simulink model "CUSTOMPID"  (R2020b)
settings: Solver=FixedStepAuto  StartTime=0.0  StopTime=2  FixedStep=0.01  RelTol=1e-3
undefined symbols (not defined in the file): cont_tf5, DiscIntNeverNeededParam, sigbuilder_block, sysConverted, tf5
settings Model: DataTypeOverride=Off  FPTShortcutValueString='{{},{''BaselineRun'',1,1,1,''BaselineRun'','''',{},''M'','''',''''},{''BaselineRun_2'',1,1,1,''BaselineRun_2'','''',{},''M'','''',''''}}'  Creator=EMRE  LastModifiedBy=EMRE
settings SolverCC: AlgebraicLoopSolver=LineSearch
settings OptimizationCC: BlockReduction=off  ConditionallyExecuteInputs=off  DefaultParameterBehavior=Inlined
settings DebuggingCC: SignalRangeChecking=warning  AlgebraicLoopMsg=error  SingleTaskRateTransMsg=error
settings HardwareCC: ProdBitPerPointer=32  ProdBitPerSizeT=32  ProdBitPerPtrDiffT=32  ProdLargestAtomicFloat=None  ProdIntDivRoundTo=Undefined  ProdEndianess=Unspecified  ProdWordSize=32  ProdHWDeviceType=ASIC/FPGA->ASIC/FPGA  TargetBitPerPointer=64  TargetBitPerSizeT=64  TargetBitPerPtrDiffT=64  TargetLongLongMode=on  TargetIntDivRoundTo=Zero  TargetEndianess=LittleEndian  TargetWordSize=64  TargetHWDeviceType=Custom Processor->MATLAB Host Computer  ProdEqTarget=off

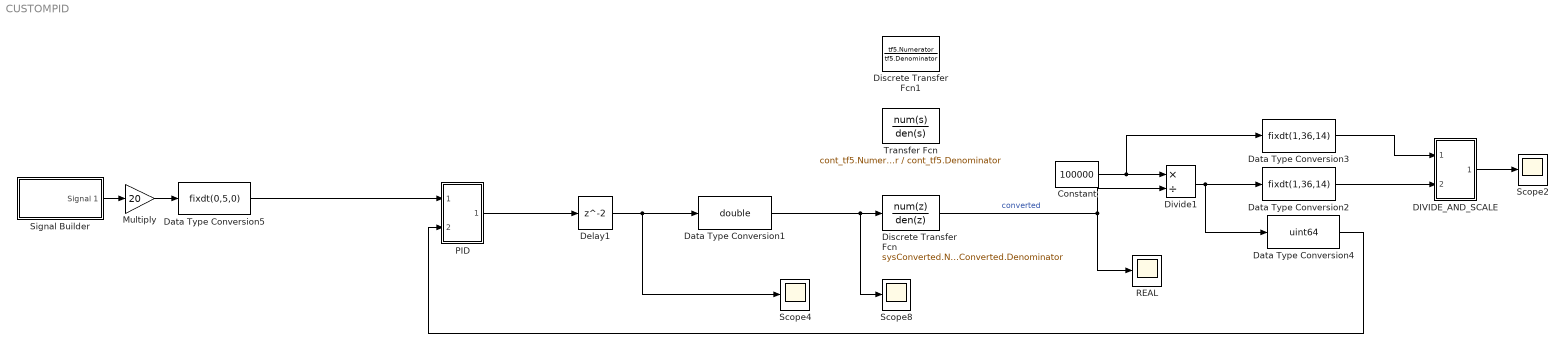
== system CUSTOMPID ==
  Constant : Constant  Value=100000
  DIVIDE_AND_SCALE : Subsystem
  Data Type Conversion1 : DataTypeConversion  OutDataTypeStr=double
  Data Type Conversion2 : DataTypeConversion  OutDataTypeStr=fixdt(1,36,14)
  Data Type Conversion3 : DataTypeConversion  OutDataTypeStr=fixdt(1,36,14)
  Data Type Conversion4 : DataTypeConversion  OutDataTypeStr=uint64  SaturateOnIntegerOverflow=on
  Data Type Conversion5 : DataTypeConversion  OutDataTypeStr=fixdt(0,5,0)
  Delay1 : Delay
  Discrete Transfer Fcn : DiscreteTransferFcn  Numerator=sysConverted.Numerator  Denominator=sysConverted.Denominator  InitialStates=1  SampleTime=0.01
  Discrete Transfer Fcn1 : DiscreteTransferFcn  Numerator=tf5.Numerator  Denominator=tf5.Denominator  SampleTime=1/100
  Divide1 : Product  Inputs=*/  RndMeth=Zero  SaturateOnIntegerOverflow=on
  Multiply : Gain  Gain=20
  PID : Subsystem
  REAL : Scope
  Scope2 : Scope
  Scope4 : Scope
  Scope8 : Scope
  Signal Builder : Subsystem  Tag=STV Subsys  LoadFcn=sigbuilder_block('load');  StartFcn=sigbuilder_block('start');  StopFcn=sigbuilder_block('stop');  ClipboardFcn=sigbuilder_block('clipboard');  mask(Sigbuilder block){tuvar=[0:10]}
      mask help: Simulink:masks:SigbuilderBlock_MD
      mask init:
      | if ~strcmp(get_param(bdroot(gcbh),'SimulationStatus'),'stopped') tuvar = sigbuilder_block('maskInit'); end
      settings: CopyFcn=sigbuilder_block('copy');  DeleteFcn=sigbuilder_block('delete');  ModelCloseFcn=sigbuilder_block('modelClose');  PreSaveFcn=sigbuilder_block('preSave');  PauseFcn=sigbuilder_block('pause');  ContinueFcn=sigbuilder_block('continue');  NameChangeFcn=sigbuilder_block('namechange');  OpenFcn=sigbuilder_block('open',[437.6 199.2 550.4 400 ]);  CloseFcn=sigbuilder_block('close');
      mask Display: plot(0, 0, 100, 100,[2, 2, 32, 32, 2], [68, 8, 8, 68, 68],[32, 2], [38, 38], [32, 19, 2],[53, 60, 44], [32, 17, 17, 2],[16, 16, 31, 31]);txt = getActiveGroup(gcbh);text(2, 100, txt,'verticalAlignment', 'top');
  Transfer Fcn : TransferFcn  Numerator=cont_tf5.Numerator  Denominator=cont_tf5.Denominator
  wires:
  Multiply/1 -> Data Type Conversion5/1
  Signal Builder/1(Signal 1) -> Multiply/1
  Discrete Transfer Fcn/1 -> REAL/1, Divide1/2  "converted"
  Data Type Conversion1/1 -> Discrete Transfer Fcn/1, Scope8/1
  Data Type Conversion2/1 -> DIVIDE_AND_SCALE/2(In2)
  Constant/1 -> Data Type Conversion3/1, Divide1/1
  DIVIDE_AND_SCALE/1(Out1) -> Scope2/1
  Data Type Conversion3/1 -> DIVIDE_AND_SCALE/1(In1)
  Divide1/1 -> Data Type Conversion4/1, Data Type Conversion2/1
  PID/1(Out1) -> Delay1/1
  Data Type Conversion5/1 -> PID/1(In1)
  Data Type Conversion4/1 -> PID/2(In2)
  Delay1/1 -> Data Type Conversion1/1, Scope4/1

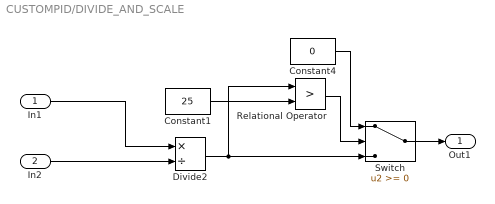
== system CUSTOMPID/DIVIDE_AND_SCALE ==
  In1 : Inport
  In2 : Inport  Port=2
  Constant1 : Constant  Value=25  OutDataTypeStr=fixdt(1,36,0)
  Constant4 : Constant  Value=0  OutDataTypeStr=fixdt(1,36,0)
  Divide2 : Product  Inputs=*/  OutMin=0  OutMax=25  OutDataTypeStr=fixdt(1,36,0)  RndMeth=Zero  SaturateOnIntegerOverflow=on
  Relational Operator : RelationalOperator  Operator=>  OutDataTypeStr=boolean  RndMeth=Simplest
  Switch : Switch  OutDataTypeStr=fixdt(1,36,0)
  Out1 : Outport
  wires:
  Switch/1 -> Out1/1
  Constant1/1 -> Relational Operator/2
  Constant4/1 -> Switch/1
  Relational Operator/1 -> Switch/2
  Divide2/1 -> Relational Operator/1, Switch/3
  In2/1 -> Divide2/2
  In1/1 -> Divide2/1

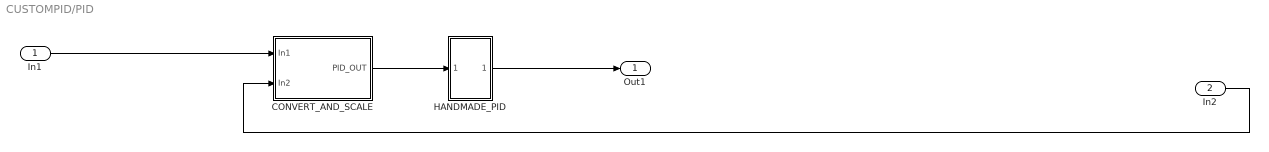
== system CUSTOMPID/PID ==
  In1 : Inport  SampleTime=1/100
  In2 : Inport  Port=2  SampleTime=1/100
  CONVERT_AND_SCALE : Subsystem
  HANDMADE_PID : Subsystem
  Out1 : Outport  SampleTime=1/100
  wires:
  CONVERT_AND_SCALE/1(PID_OUT) -> HANDMADE_PID/1(PID_OUT)
  HANDMADE_PID/1(Out1) -> Out1/1
  In1/1 -> CONVERT_AND_SCALE/1(In1)
  In2/1 -> CONVERT_AND_SCALE/2(In2)

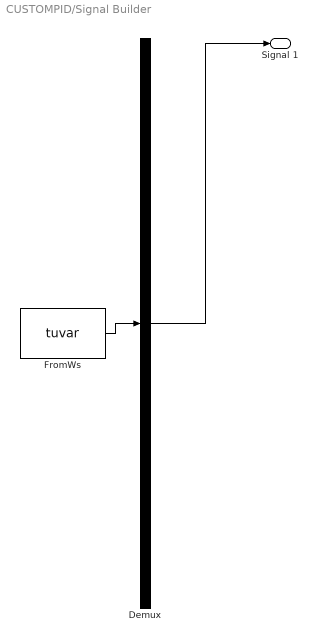
== system CUSTOMPID/Signal Builder ==
  Demux : Demux  Tag=STV Demux  Outputs=1
      settings: DisplayOption=none
  FromWs : FromWorkspace  Tag=STV FromWs  VariableName=tuvar
      SigBuilderData=|
      | common.afterFinalStr = 'Extrapolate'
      | common.sampleTime = 0
      | dataSet.timeRange = [0 2]
      | dataSet.name = 'Group 1'
      | sbobj.Groups.Name = 'Group 1'
      | sbobj.Groups.Signals.Name = 'Signal 1'
      | sbobj.Groups.Signals.XData = [0 0.2 0.5 0.7 0.7 1 1 1.1 1.1 1.3 1.3 1.4 1.4 1.5 1.5 1.7 1.7 2]
      | sbobj.Groups.Signals.YData = [1 1 1 1 0.2 0.195 0.99 0.99 0.2 0.2 0 0 0.4 0.4 0 0 1 1]
      | sbobj.Groups.TimeRange = [0 2]
  Signal 1 : Outport  Tag=STV Outport
  wires:
  Demux/1 -> Signal 1/1
  FromWs/1 -> Demux/1

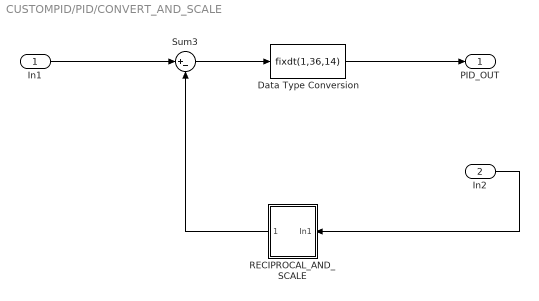
== system CUSTOMPID/PID/CONVERT_AND_SCALE ==
  In1 : Inport  SampleTime=1/100
  In2 : Inport  Port=2  SampleTime=1/100
  Data Type Conversion : DataTypeConversion  OutDataTypeStr=fixdt(1,36,14)
  RECIPROCAL_AND_SCALE : Subsystem
  Sum3 : Sum  Inputs=|+-
  PID_OUT : Outport  SampleTime=1/100
  wires:
  In1/1 -> Sum3/1
  RECIPROCAL_AND_SCALE/1(Out1) -> Sum3/2
  In2/1 -> RECIPROCAL_AND_SCALE/1(In1)
  Data Type Conversion/1 -> PID_OUT/1
  Sum3/1 -> Data Type Conversion/1

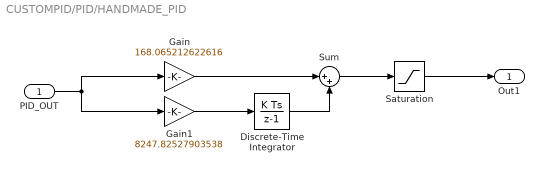
== system CUSTOMPID/PID/HANDMADE_PID ==
  PID_OUT : Inport  OutMin=-25  OutMax=25  OutDataTypeStr=fixdt(1,36,14)  SampleTime=1/100
  Discrete-Time Integrator : DiscreteIntegrator  InitialCondition=1  SampleTime=1/100  OutDataTypeStr=fixdt(1,36,14)  ICPrevOutput=DiscIntNeverNeededParam  ICPrevScaledInput=DiscIntNeverNeededParam
  Gain : Gain  Gain=168.065212622616  OutDataTypeStr=fixdt(1,36,14)
  Gain1 : Gain  Gain=8247.82527903538  OutDataTypeStr=fixdt(1,36,14)
  Saturation : Saturate  UpperLimit=10000  LowerLimit=0
  Sum : Sum  Inputs=|++  OutDataTypeStr=fixdt(1,36,14)
  Out1 : Outport  OutMin=0  OutMax=10000  SampleTime=1/100
  wires:
  PID_OUT/1 -> Gain1/1, Gain/1
  Gain/1 -> Sum/1
  Discrete-Time Integrator/1 -> Sum/2
  Gain1/1 -> Discrete-Time Integrator/1
  Sum/1 -> Saturation/1
  Saturation/1 -> Out1/1

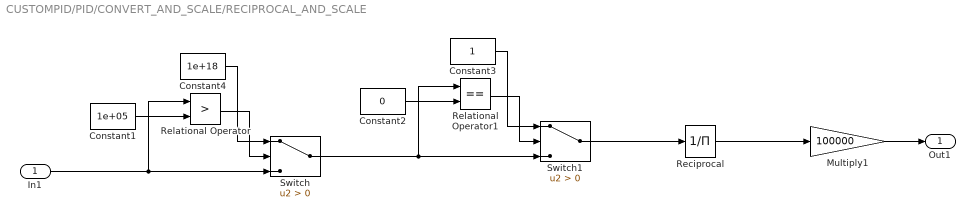
== system CUSTOMPID/PID/CONVERT_AND_SCALE/RECIPROCAL_AND_SCALE ==
  In1 : Inport  SampleTime=1/100
  Constant1 : Constant  Value=1e+05  OutDataTypeStr=fixdt(1,64,0)  SampleTime=1/100
  Constant2 : Constant  Value=0  OutDataTypeStr=fixdt(1,64,0)  SampleTime=1/100
  Constant3 : Constant  VectorParams1D=off  OutMin=0  OutDataTypeStr=fixdt(1,64,0)  SampleTime=1/100
  Constant4 : Constant  Value=1e+18  OutDataTypeStr=fixdt(1,64,0)  SampleTime=1/100
  Multiply1 : Gain  Gain=100000  OutDataTypeStr=fixdt(1,36,14)
  Reciprocal : Product  Inputs=/  OutMax=31  OutDataTypeStr=fixdt(1,36,30)  RndMeth=Zero  SaturateOnIntegerOverflow=on
  Relational Operator : RelationalOperator  Operator=>  OutDataTypeStr=boolean  RndMeth=Simplest
  Relational Operator1 : RelationalOperator  Operator===  OutDataTypeStr=boolean  RndMeth=Simplest
  Switch : Switch  Criteria=u2 > Threshold  OutDataTypeStr=fixdt(1,64,0)
  Switch1 : Switch  Criteria=u2 > Threshold  OutDataTypeStr=fixdt(1,64,0)
  Out1 : Outport  SampleTime=1/100
  wires:
  In1/1 -> Switch/3, Relational Operator/1
  Relational Operator/1 -> Switch/2
  Reciprocal/1 -> Multiply1/1
  Constant4/1 -> Switch/1
  Constant1/1 -> Relational Operator/2
  Multiply1/1 -> Out1/1
  Constant2/1 -> Relational Operator1/2
  Switch/1 -> Switch1/3, Relational Operator1/1
  Relational Operator1/1 -> Switch1/2
  Constant3/1 -> Switch1/1
  Switch1/1 -> Reciprocal/1
